simulink model "ukol_1_a_se_sumem"  (R2017a)
settings: Solver=VariableStepAuto  StartTime=0.0  StopTime=100  MaxStep=1e-2  RelTol=1e-3  EnableMultiTasking=on
libraries: simulink x2, cstblocks x1
settings Model: Creator=kuhaj  LastModifiedBy=tomas
settings DataIOCC: LimitDataPoints=on
settings OptimizationCC: LifeSpan=inf
settings DebuggingCC: AllowSymbolicDim=off  SFUnexpectedBacktrackingDiag=warning  SFNoUnconditionalDefaultTransitionDiag=warning  SFExecutionAtInitializationDiag=none
settings ModelReferenceCC: PropagateSignalLabelsOutOfModel=off
settings GRTTargetCC: TargetLangStandard=C89/C90 (ANSI)
settings ConfigComp: CovMetricSettings=dw  CovHtmlReporting=on  CovSaveCumulativeToWorkspaceVar=on  CovSaveSingleToWorkspaceVar=on  CovExternalEMLEnable=off

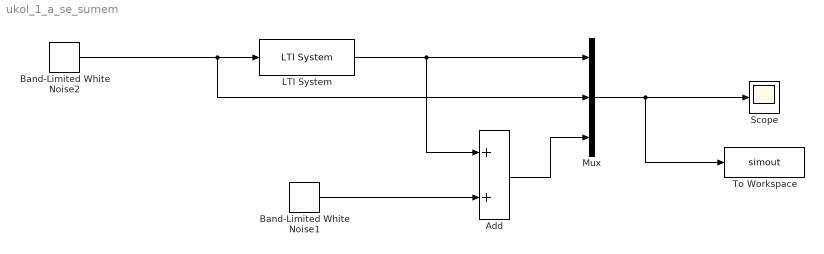
== system ukol_1_a_se_sumem ==
  Add : Sum
  Band-Limited White Noise1 : simulink/Sources/Band-Limited White Noise  Cov=[0.01]  Ts=0.2  seed=[23341]
  Band-Limited White Noise2 : simulink/Sources/Band-Limited White Noise  Cov=[1]  Ts=0.2  seed=[23341]
  LTI System : cstblocks/LTI System  sys=discrete_Fs  IC=[]
  Mux : Mux  Inputs=3
  Scope : Scope
  To Workspace : ToWorkspace  VariableName=simout  SaveFormat=Timeseries  SampleTime=-1
  wires:
  Mux/1 -> To Workspace/1, Scope/1
  Add/1 -> Mux/3
  Band-Limited White Noise2/1 -> LTI System/1, Mux/2
  Band-Limited White Noise1/1 -> Add/2
  LTI System/1 -> Add/1, Mux/1
